simulink model "E_Platoon_simscape"  (R2025b)
settings: Solver=FixedStepAuto  StartTime=0.0  StopTime=inf  FixedStep=0.01  RelTol=1e-3
values from neighbouring files (symbols this model uses):
  battery_SOC_resistance = battery_SOC(:,3)    [EV_Truck.m]
  battery_SOC_SOC = battery_SOC(:,1)    [EV_Truck.m]
  battery_SOC_voltage = battery_SOC(:,2)    [EV_Truck.m]
  motor_efficiency_efficiency = table2array(motor_efficiency(2:height(motor_efficiency),2:width(motor_efficiency)))    [EV_Truck.m]
  motor_efficiency_RPM = table2array(motor_efficiency(2:height(motor_efficiency),1))    [EV_Truck.m]
  motor_efficiency_torque = transpose(motor_efficiency_torque)    [EV_Truck.m]
  motor_RPM_torque = table2array(motor_torque(1:14,1))    [EV_Truck.m]
  motor_torque_RPM = table2array(motor_torque(1:14,2))    [EV_Truck.m]
undefined symbols (not defined in the file or in its folder): battery_builder_rtmsupport, DiscIntNeverNeededParam, gcbh
libraries: simulink x8, fl_lib x8, nesl_utility x8, Batteries_lib x4, mpcadaslib x2, slpidlib x2
(part 3 of 3)

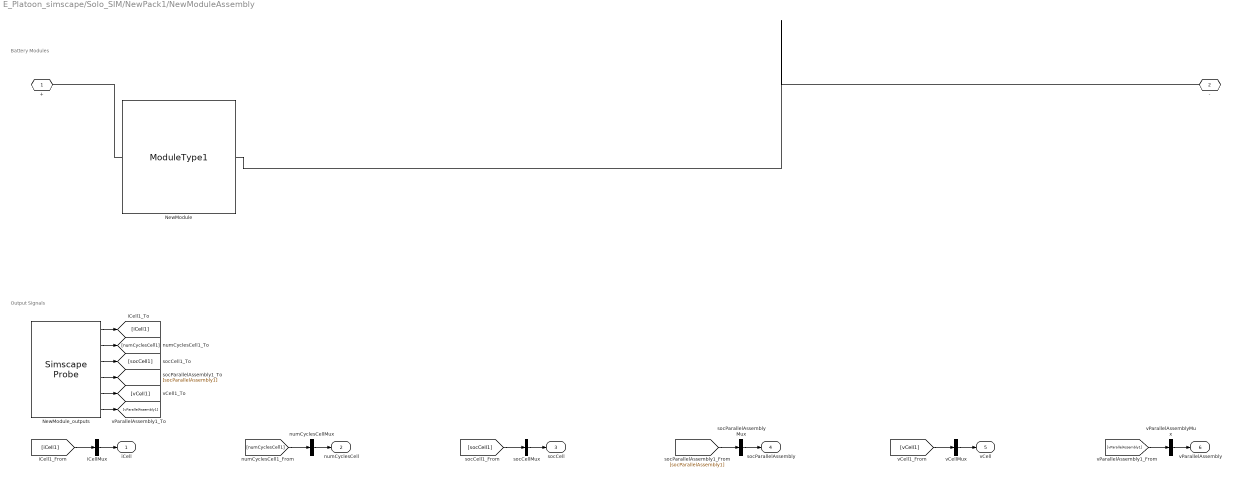
== system E_Platoon_simscape/Solo_SIM/NewPack1/NewModuleAssembly ==
  note: Output Signals
  note: Battery Modules
  NewModule : Batteries_lib/Modules/ModuleType1  SOC_vecCell=[0, .01, .02, .03, .04, .05, .06, .07, .08, .09, .1, .11, .12, .13, .14, .15, .16, .17, .18, .19, .2, .21, .22, .23, .24, .25, .26, .27, .28, .29, .3, .31, .32, .33, .34, .35, .36, .37, .38, .39, .4, .41, .42, .43, .44, .45, .46, .47, .48, .49, .5, .51, .52, .53, .54, .55, .56, .57, .58, .59, .6, .61, .62, .63, .64, .65, .66, .67, .68, .69, .7, .71, .72, .73, .74, .75, .76, .77, .78, .79, .8, .81, .82, .83, .84, .85, .86, .87, .88, .89, .9, .91, .92, .93, .94, .95, .96, .97, .98, .99, 1]  V0_vecCell=[35.84591, 36.10202, 36.35814, 36.61425, 36.87037, 37.12649, 37.3826, 37.63872, 37.89483, 38.09951, 38.20904, 38.28916, 38.37306, 38.42308, 38.45482, 38.47744, 38.49779, 38.54815, 38.5883, 38.63829, 38.68732, 38.72975, 38.77111, 38.80795, 38.83724, 38.8617, 38.89023, 38.9273, 38.96054, 38.98786, 39.01519, 39.03864, 39.06385, 39.08223, 39.1006, 39.11898, 39.13735, 39.15508, 39.16412, 39.17437, 39.18528, 39.19619, 39.20709, 39.21696, 39.22232, 39.22753, 39.23277, 39.23672, 39.23942, 39.24211, 39.24481, 39.24786, 39.25094, 39.2539, 39.25686, 39.26099, 39.26708, 39.27551, 39.28394, 39.29233, 39.30067, 39.31557, 39.33487, 39.35402, 39.37113, 39.38825, 39.40815, 39.43406, 39.46187, 39.48968, 39.51913, 39.55031, 39.5817, 39.60619, 39.62271, 39.63907, 39.65521, 39.67134, 39.68137, 39.69071, 39.70005, 39.7052, 39.70868, 39.70916, 39.70862, 39.70807, 39.70752, 39.71037, 39.72142, 39.72908, 39.73651, 39.73911, 39.73577, 39.72919, 39.73278, 39.7392, 39.74638, 39.75462, 39.8136, 40.01141, 40.30627] V  V_rangeCell=[27, Inf] V  R0_vecCell=[.47635, .41138, .35007, .29417, .24882, .2142, .18886, .17031, .1569, .14398, .13028, .11716, .10632, .09512, .08414, .07347, .06467, .05964, .05477, .05154, .04841, .04625, .04448, .04297, .04112, .03908, .0378, .03771, .03746, .03699, .03652, .03598, .03587, .03552, .03517, .03481, .03446, .03417, .03358, .03336, .03321, .03305, .0329, .0327, .03227, .03186, .03148, .03105, .03058, .03011, .02964, .02918, .02875, .02834, .02792, .02762, .02745, .02737, .02729, .02722, .02715, .0274, .02786, .0283, .02854, .02877, .02906, .02956, .03013, .0307, .03135, .03204, .03271, .03308, .03307, .03314, .03323, .03332, .03312, .03288, .03264, .03224, .03172, .03113, .03057, .03001, .02945, .02905, .02924, .0293, .02938, .02923, .02879, .02803, .02792, .02793, .02786, .02652, .02587, .02701, .00941] Ohm  AHCell=50.41 A*hr  extrapolation_optionCell=simscape.enum.extrapolation.nearest  P=18  S=18  iCell_specify=off  iCell_priority=None  iCell=0 A  iCell_nominal_specify=off  iCell_nominal_value=1  iCell_nominal_unit=A  vCell_specify=off  vCell_priority=None  vCell=0 V  vCell_nominal_specify=off  vCell_nominal_value=1  vCell_nominal_unit=V  socCell_specify=off  socCell_priority=High  socCell=1  socCell_nominal_specify=off  socCell_nominal_value=1  socCell_nominal_unit=1  numCyclesCell_specify=off  numCyclesCell_priority=High  numCyclesCell=0  numCyclesCell_nominal_specify=off  numCyclesCell_nominal_value=1  numCyclesCell_nominal_unit=1  vParallelAssembly_specify=off  vParallelAssembly_priority=None  vParallelAssembly=repmat(0, 18, 1) V  vParallelAssembly_nominal_specify=off  vParallelAssembly_nominal_value=1  vParallelAssembly_nominal_unit=V  socParallelAssembly_specify=off  socParallelAssembly_priority=None  socParallelAssembly=repmat(1, 18, 1)  socParallelAssembly_nominal_specify=off  socParallelAssembly_nominal_value=1  socParallelAssembly_nominal_unit=1
      settings: InternalSimscapePortConfiguration="{\"Bottom\":[{\"id\":\"n\",\"label\":\"-\",\"type\":\"foundation.electrical.electrical\"}],\"Left\":[],\"Right\":[],\"Top\":[{\"id\":\"p\",\"label\":\"+\",\"type\":\"foundation.electrical.electrical\"}]}"
  NewModule_outputs : SimscapeProbe  BoundBlock=10972  Variables="{\"iCell\":{\"Unit\":\"A\",\"PortLabel\":\"iCell\",\"Probing\":\"ON\"},\"numCyclesCell\":{\"Unit\":\"1\",\"PortLabel\":\"numCyclesCell\",\"Probing\":\"ON\"},\"socCell\":{\"Unit\":\"1\",\"PortLabel\":\"socCell\",\"Probing\":\"ON\"},\"socParallelAssembly\":{\"Unit\":\"1\",\"PortLabel\":\"socParallelAssembly\",\"Probing\":\"ON\"},\"vCell\":{\"Unit\":\"V\",\"PortLabel\":\"vCell\",\"Probing\":\"ON\"},\"vParallelAssembly\":{\"Unit\":\"V\",\"PortLabel\":\"vParallelAssembly\",\"Probing\":\"ON\"}}"
  iCellMux : Mux  Inputs=1
  numCyclesCellMux : Mux  Inputs=1
  socCellMux : Mux  Inputs=1
  socParallelAssemblyMux : Mux  Inputs=1
  vCellMux : Mux  Inputs=1
  vParallelAssemblyMux : Mux  Inputs=1
  + : PMIOPort  Side=Left
  - : PMIOPort  Port=2  Side=Right
  iCell : Outport
  numCyclesCell : Outport  Port=2
  socCell : Outport  Port=3
  socParallelAssembly : Outport  Port=4
  vCell : Outport  Port=5
  vParallelAssembly : Outport  Port=6
  wires:
  [vParallelAssembly1] -> vParallelAssemblyMux/1
  vParallelAssemblyMux/1 -> vParallelAssembly/1
  NewModule_outputs/6 -> [vParallelAssembly1]
  [vCell1] -> vCellMux/1
  vCellMux/1 -> vCell/1
  NewModule_outputs/5 -> [vCell1]
  [socParallelAssembly1] -> socParallelAssemblyMux/1
  socParallelAssemblyMux/1 -> socParallelAssembly/1
  NewModule_outputs/4 -> [socParallelAssembly1]
  [socCell1] -> socCellMux/1
  socCellMux/1 -> socCell/1
  NewModule_outputs/3 -> [socCell1]
  [numCyclesCell1] -> numCyclesCellMux/1
  numCyclesCellMux/1 -> numCyclesCell/1
  NewModule_outputs/2 -> [numCyclesCell1]
  [iCell1] -> iCellMux/1
  iCellMux/1 -> iCell/1
  NewModule_outputs/1 -> [iCell1]
  connections:
  NewModule/RConn1 -- -/RConn1
  NewModule/LConn1 -- +/RConn1

== matlab function E_Platoon_simscape/Solo_SIM/MATLAB Function ==
  data: P input; OCV input; R0 input; I output
function I = current_from_power(P, OCV, R0)
% 1-R battery model:
%   Vt = OCV - R0*I
%   P  = Vt*I = I*(OCV - R0*I)
% => R0*I^2 - OCV*I + P = 0
%   I = (OCV - sqrt(OCV^2 - 4*R0*P)) / (2*R0)
%
%   P>0 -> I>0 (discharge)
%   P<0 -> I<0 (regen/charge)

epsR = 1e-12;
epsV = 1e-6;
R0  = max(R0, epsR);
OCV = max(OCV, epsV);

% Discriminant
D = OCV*OCV - 4*R0*P;

% If D < 0, the requested P is infeasible under this simple model.
% Clamp to 0 to avoid complex values (simple fallback).
if D < 0
    D = 0;
end

% Minus-branch current
I = (OCV - sqrt(D)) / (2*R0);

% Safety
if ~isfinite(I)
    I = 0;
end
end

== matlab function E_Platoon_simscape/LV_SIM/MATLAB Function ==
  data: P input; OCV input; R0 input; I output
function I = current_from_power(P, OCV, R0)
% 1-R battery model:
%   Vt = OCV - R0*I
%   P  = Vt*I = I*(OCV - R0*I)
% => R0*I^2 - OCV*I + P = 0
%   I = (OCV - sqrt(OCV^2 - 4*R0*P)) / (2*R0)
%
%   P>0 -> I>0 (discharge)
%   P<0 -> I<0 (regen/charge)

epsR = 1e-12;
epsV = 1e-6;
R0  = max(R0, epsR);
OCV = max(OCV, epsV);

% Discriminant
D = OCV*OCV - 4*R0*P;

% If D < 0, the requested P is infeasible under this simple model.
% Clamp to 0 to avoid complex values (simple fallback).
if D < 0
    D = 0;
end

% Minus-branch current
I = (OCV - sqrt(D)) / (2*R0);

% Safety
if ~isfinite(I)
    I = 0;
end
end

== matlab function E_Platoon_simscape/FV1_SIM/MATLAB Function ==
  data: P input; OCV input; R0 input; I output
function I = current_from_power(P, OCV, R0)
% 1-R battery model:
%   Vt = OCV - R0*I
%   P  = Vt*I = I*(OCV - R0*I)
% => R0*I^2 - OCV*I + P = 0
%   I = (OCV - sqrt(OCV^2 - 4*R0*P)) / (2*R0)
%
%   P>0 -> I>0 (discharge)
%   P<0 -> I<0 (regen/charge)

epsR = 1e-12;
epsV = 1e-6;
R0  = max(R0, epsR);
OCV = max(OCV, epsV);

% Discriminant
D = OCV*OCV - 4*R0*P;

% If D < 0, the requested P is infeasible under this simple model.
% Clamp to 0 to avoid complex values (simple fallback).
if D < 0
    D = 0;
end

% Minus-branch current
I = (OCV - sqrt(D)) / (2*R0);

% Safety
if ~isfinite(I)
    I = 0;
end
end

== matlab function E_Platoon_simscape/FV1_SIM/ACC system/MATLAB Function ==
  data: accel input; acceleration output
function acceleration  = fcn(accel)

if accel > 0 
    acceleration = (accel * 100)/0.15;
elseif accel < 0 
    acceleration = (accel * 100)/0.33;
else
    acceleration = 0; % accel이 0이거나 NaN일 경우에도 대응
end

== matlab function E_Platoon_simscape/FV1_SIM/Drag coefficient ==
  data: IVD input; C_drag output
function C_drag = fcn(IVD)
a = -0.4629;
b = -0.068;
c = 0.6441;

C_drag = a * exp(b * (IVD-8)) + c;

== matlab function E_Platoon_simscape/FV2_SIM/ACC system/MATLAB Function ==
  data: accel input; acceleration output
function acceleration  = fcn(accel)

if accel > 0 
    acceleration = (accel * 100)/0.15;
elseif accel < 0 
    acceleration = (accel * 100)/0.33;
else
    acceleration = 0; % accel이 0이거나 NaN일 경우에도 대응
end

== matlab function E_Platoon_simscape/FV2_SIM/Drag coefficient ==
  data: IVD input; C_drag output
function C_drag = fcn(IVD)
a = -0.4629;
b = -0.068;
c = 0.6441;

C_drag = a * exp(b * (IVD-8)) + c;

== matlab function E_Platoon_simscape/LV_SIM/Drag coefficient1 ==
  data: IVD input; C_drag output
function C_drag = fcn(IVD)
a = -0.1012;
b = -0.1002;
c = 0.6441;

C_drag = a * exp(b * (IVD-8)) + c;

== matlab function E_Platoon_simscape/FV2_SIM/MATLAB Function ==
  data: P input; OCV input; R0 input; I output
function I = current_from_power(P, OCV, R0)
% 1-R battery model:
%   Vt = OCV - R0*I
%   P  = Vt*I = I*(OCV - R0*I)
% => R0*I^2 - OCV*I + P = 0
%   I = (OCV - sqrt(OCV^2 - 4*R0*P)) / (2*R0)
%
%   P>0 -> I>0 (discharge)
%   P<0 -> I<0 (regen/charge)

epsR = 1e-12;
epsV = 1e-6;
R0  = max(R0, epsR);
OCV = max(OCV, epsV);

% Discriminant
D = OCV*OCV - 4*R0*P;

% If D < 0, the requested P is infeasible under this simple model.
% Clamp to 0 to avoid complex values (simple fallback).
if D < 0
    D = 0;
end

% Minus-branch current
I = (OCV - sqrt(D)) / (2*R0);

% Safety
if ~isfinite(I)
    I = 0;
end
end
